simulink model "Levant"  (R2023a)
settings: Solver=ode45  StartTime=0.0  StopTime=10.0  FixedStep=0.0001  RelTol=1e-3
undefined symbols (not defined in the file or in its folder): sigbuilder_block
settings Model: Creator=headl  LastModifiedBy=headl
settings SolverCC: InitialStep=.01  AlgebraicLoopSolver=TrustRegion
settings DebuggingCC: UnconnectedInputMsg=warning  UnconnectedOutputMsg=warning  UnconnectedLineMsg=warning
settings ModelReferenceCC: EnableRefExpFcnMdlSchedulingChecks=on
settings SFSimCC: CustomCodeUndefinedFunction=UseInterfaceOnly

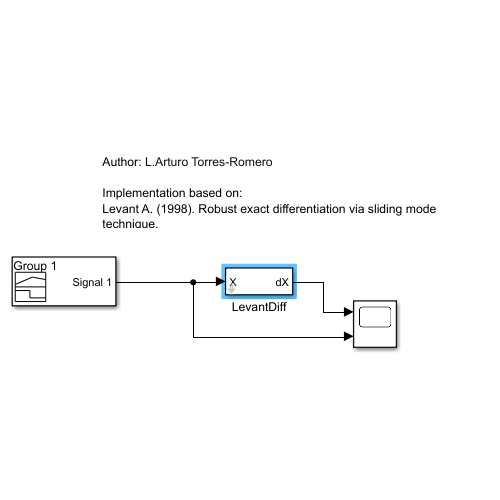
[thumbnail: Simulink's stored preview of the top-level diagram]
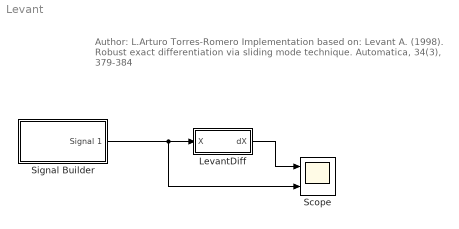
== system Levant ==
  note: Author: L.Arturo Torres-Romero
      |
      | Implementation based on:
      | Levant A. (1998). Robust exact differentiation via sliding mode technique.
      | Automatica, 34(3), 379-384
  LevantDiff : Subsystem  mask{lambda1=60, alpha1=2000}
      mask prompts: lambda1 "Lambda :"; alpha1 "Alpha    :"
      mask help: Levant differenciator
      mask Help: This is based on Levant A. (1998). Robust exact differentiation via sliding mode technique. Automatica, 34(3), 379-384
  Scope : Scope  NumInputPorts=2
  Signal Builder : Subsystem  Tag=STV Subsys  LoadFcn=sigbuilder_block('load');  StartFcn=sigbuilder_block('start');  StopFcn=sigbuilder_block('stop');  ClipboardFcn=sigbuilder_block('clipboard');  mask(Sigbuilder block){tuvar=[0:10]}
      mask help: Simulink:masks:SigbuilderBlock_MD
      mask init:
      | if ~strcmp(get_param(bdroot(gcbh),'SimulationStatus'),'stopped') tuvar = sigbuilder_block('maskInit'); end
      settings: CopyFcn=sigbuilder_block('copy');  DeleteFcn=sigbuilder_block('delete');  ModelCloseFcn=sigbuilder_block('modelClose');  PreSaveFcn=sigbuilder_block('preSave');  PauseFcn=sigbuilder_block('pause');  ContinueFcn=sigbuilder_block('continue');  NameChangeFcn=sigbuilder_block('namechange');  OpenFcn=sigbuilder_block('open',[5.4 30 1141.2 522.6 ]);  CloseFcn=sigbuilder_block('close');
      mask Display: plot(0, 0, 100, 100,[2, 2, 32, 32, 2], [68, 8, 8, 68, 68],[32, 2], [38, 38], [32, 19, 2],[53, 60, 44], [32, 17, 17, 2],[16, 16, 31, 31]);txt = getActiveGroup(gcbh);text(2, 100, txt,'verticalAlignment', 'top');
  wires:
  Signal Builder/1(Signal 1) -> LevantDiff/1(X), Scope/2
  LevantDiff/1(dX) -> Scope/1

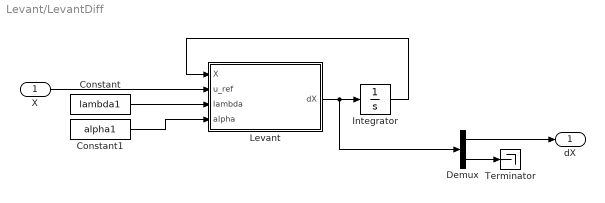
== system Levant/LevantDiff ==
  X : Inport
  Constant : Constant  Value=lambda1
  Constant1 : Constant  Value=alpha1
  Demux : Demux  Outputs=2
  Integrator : Integrator  InitialCondition=[0 0]
  Levant : MATLAB Function  TreatAsAtomicUnit=on
  Terminator : Terminator
  dX : Outport  VectorParamsAs1DForOutWhenUnconnected=off
  wires:
  X/1 -> Levant/2(u_ref)
  Levant/1(dX) -> Integrator/1, Demux/1
  Integrator/1 -> Levant/1(X)
  Constant/1 -> Levant/3(lambda)
  Constant1/1 -> Levant/4(alpha)
  Demux/1 -> dX/1
  Demux/2 -> Terminator/1

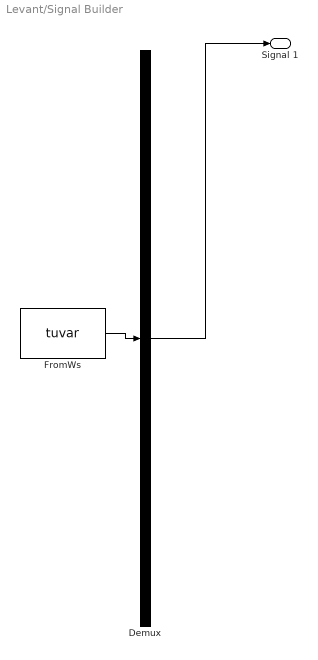
== system Levant/Signal Builder ==
  Demux : Demux  Tag=STV Demux  Outputs=1
      settings: DisplayOption=none
  FromWs : FromWorkspace  Tag=STV FromWs  VariableName=tuvar
      SigBuilderData=|
      | common.afterFinalStr = 'Extrapolate'
      | common.sampleTime = 0
      | dataSet.timeRange = [0 10]
      | dataSet.name = 'Group 1'
      | sbobj.Groups.Name = 'Group 1'
      | sbobj.Groups.Signals.Name = 'Signal 1'
      | sbobj.Groups.Signals.XData = [0 0.0200400801603 0.0400801603206 0.060120240481 0.0801603206413 0.100200400802 0.120240480962 0.140280561122 0.160320641283 0.180360721443 0.200400801603 0.220440881764 ... (500 elements, 1x500)]
      | sbobj.Groups.Signals.YData = [0 0.0125912209985 0.0251804457201 0.0377656782048 0.050344923125 0.0629161861029 0.0754774740258 0.0880267953628 0.10056216048 0.113081581956 0.125583074899 0.138064657256 ... (500 elements, 1x500)]
  Signal 1 : Outport  Tag=STV Outport  VectorParamsAs1DForOutWhenUnconnected=off
  wires:
  Demux/1 -> Signal 1/1
  FromWs/1 -> Demux/1

== matlab function Levant/LevantDiff/Levant ==
  data: dX output; X input; u_ref input; lambda input; alpha input
%*************************************************
% Author: L.Arturo Torres-Romero
% based on 
% Levant A. (1998). Robust exact differentiation via sliding mode technique. 
% Automatica, 34(3), 379-384
%*************************************************

function dX = LevantDiff(X, u_ref, lambda, alpha) 
z_0=X(1);    z_1= X(2); 

 
%Levant differenciator
 d_z_0=z_1-lambda*sqrt(abs(z_0-u_ref))*sign(z_0-u_ref);
 d_z_1=-alpha*sign(z_0-u_ref);
      
dX = [d_z_0;d_z_1];
end
